simulink model "Target_Control_System"  (R2021b)
settings: Solver=FixedStepDiscrete  StartTime=0.0  StopTime=5  RelTol=1e-3
PreLoadFcn:
  | RTWConfigurationCB('preloadfcn', bdroot);
PostLoadFcn:
  | load('configuration/data_struct.mat');
  | load('configuration/fluxMaps_propMotor.mat');
  | load('configuration/parameterInit_PROP.mat');
  | load('configuration/parameterInit_PUMP.mat');
  | load('configuration/parameterInit_PITCH.mat');
  | load('configuration/parameterInit_TILT.mat');
  | %load('configuration/base_workspace_signal_definition.mat');
  | %load('resolvedatastores_to_baseworkspace_for_faster_simulation.mat');
model workspace (MAT data in the model file):
  SIMULATION_OPTIONS : Simulink.Parameter (value not decoded)
  TARGET_CODE_GEN : Simulink.Parameter (value not decoded)
  TCS_SAMPLE_FREQ_HZ : Simulink.Parameter (value not decoded)
symbols that are objects in the model workspace (value not decoded): TARGET_CODE_GEN, TCS_SAMPLE_FREQ_HZ
undefined symbols (not defined in the file): A_DQ_REF_LPF_INIT__PITCH, A_DQ_REF_LPF_INIT__PROP, A_DQ_REF_LPF_INIT__PUMP, A_DQ_REF_LPF_INIT__TILT, A_OBSERVER_CONFIDENCE_INIT__PITCH, A_OBSERVER_CONFIDENCE_INIT__PROP, A_OBSERVER_CONFIDENCE_INIT__PUMP, A_OBSERVER_CONFIDENCE_INIT__TILT, ACTUATOR_MAX_ANGLE_TRIP__PITCH, ACTUATOR_MIN_ANGLE_TRIP__PITCH, ACTUATOR_POS_SENSOR_INV_DIRECTION__PITCH, ACTUATOR_POS_SENSOR_INV_DIRECTION__TILT, ACTUATOR_POS_SENSOR_OFFSET__PITCH, ACTUATOR_POS_SENSOR_OFFSET__TILT, ADC_scaler1_baseaddr_TILT, ADC_SCALER_FLOAT_TO_FIXPOINT_EXPANSION, ANGLE_ELEC_FROM_SENSOR_OFFSET_INIT__PITCH, ANGLE_ELEC_FROM_SENSOR_OFFSET_INIT__PROP, ANGLE_ELEC_FROM_SENSOR_OFFSET_INIT__PUMP, ANGLE_ELEC_FROM_SENSOR_OFFSET_INIT__TILT, AUTO_CLEAR_FAULTS_ENABLED__PITCH, AUTO_CLEAR_FAULTS_ENABLED__PROP, AUTO_CLEAR_FAULTS_ENABLED__PUMP, AUTO_CLEAR_FAULTS_ENABLED__TILT, AUTO_CLEAR_FAULTS_WAIT_TICKS__PITCH, AUTO_CLEAR_FAULTS_WAIT_TICKS__PROP, AUTO_CLEAR_FAULTS_WAIT_TICKS__PUMP, AUTO_CLEAR_FAULTS_WAIT_TICKS__TILT, AUTO_I_ZERO_IDLE_TICKS__PITCH, AUTO_I_ZERO_IDLE_TICKS__PROP, AUTO_I_ZERO_IDLE_TICKS__PUMP, AUTO_I_ZERO_IDLE_TICKS__TILT, AUTO_I_ZERO_OFFSET_IDC_THRESHOLD__PITCH, AUTO_I_ZERO_OFFSET_IDC_THRESHOLD__PROP, AUTO_I_ZERO_OFFSET_IDC_THRESHOLD__PUMP, AUTO_I_ZERO_OFFSET_IDC_THRESHOLD__TILT, AUTO_I_ZERO_OFFSET_IPH_THRESHOLD__PITCH, AUTO_I_ZERO_OFFSET_IPH_THRESHOLD__PROP, AUTO_I_ZERO_OFFSET_IPH_THRESHOLD__PUMP, AUTO_I_ZERO_OFFSET_IPH_THRESHOLD__TILT, AUTO_SENSORLESS_SWITCHOVER_DISABLE_OMEGA, AUTO_SENSORLESS_SWITCHOVER_ENABLE_OMEGA, AUTO_SENSORLESS_SWITCHOVER_MIN_CONFIDENCE, AUXILIARY_PROTECTION_UNIT_BASEADDR__TILT, blanking_max_error_omega_INIT_PITCH, blanking_max_error_omega_INIT_TILT, blanking_max_error_position_INIT_PITCH, blanking_max_error_position_INIT_TILT, BRUTE_START_I_Q_REF_RAMP_SPEED__PITCH, BRUTE_START_I_Q_REF_RAMP_SPEED__PROP, BRUTE_START_I_Q_REF_RAMP_SPEED__PUMP, BRUTE_START_I_Q_REF_RAMP_SPEED__TILT, CONTROL_LOOP_DT_INIT__PITCH, CONTROL_LOOP_DT_INIT__PROP, CONTROL_LOOP_DT_INIT__PUMP, CONTROL_LOOP_DT_INIT__TILT, CORRECTION_FILTER_SCALE__PITCH, CORRECTION_FILTER_SCALE__PROP, CORRECTION_FILTER_SCALE__PUMP, CORRECTION_FILTER_SCALE__TILT ... (+458)
libraries: simulink x178, Reusables_Lib x24
(part 44 of 47)

== stateflow chart Target_Control_System/MainLoop/tiltMotor_mainLoop/Decimation gate for 10 Hz Tilt/Idle-Loop State Machine Tilt ==
  state InitialState
  state State_90
    //startup delay
    state Wait_Ticks_
    state Startup_Delay_
      entry:
      oTilt.oMot_.oState_.uiDriveState_ = 95;
      oTilt.oMot_.oOut_.uiLastFaultState_ = 0;
    (default) -> State_90.Wait_Ticks_
    State_90.Wait_Ticks_ -> Startup_Delay_ : [after(35, tick)]
  state State_246
    // Second phase of voltage nulling
    state Wait_uiDelayTicks_
    state Next
      entry:
      oTilt.oMot_.oState_.uiDriveState_ = 100;
      oTilt.oMot_.oOut_.uiEnableGateDrive_ = 0x0;
      oTilt.oMot_.oIn_.uiVoltageOffsetNullingActive_ = 0;
    (default) -> State_246.Wait_uiDelayTicks_
    State_246.Wait_uiDelayTicks_ -> State_246.Next : [after(25, tick)]
  state State_95
    // Current offset nulling
    state Wait_Ticks_
    state Current_offset_nulling
      entry:
      oTilt.oMot_.oState_.uiCurrentOffsetNullingPerformed_++;
      oTilt.oMot_.oIn_.uiCurrentOffsetNullingActive_ = 0;
      oTilt.oMot_.oIn_.uiVoltageOffsetNullingActive_ = 0;
      oTilt.oMot_.oState_.uiDriveState_ = 99;
      //SZ: still need to re-write the FPGA protection to enable the sum of current detection for fault 1034
    (default) -> State_95.Wait_Ticks_
    State_95.Wait_Ticks_ -> Current_offset_nulling : [after(6, tick)]
  state State_245
    // Initial phase of voltage nulling
    state Wait_uiDelayTicks_
    state Next
      entry:
      oTilt.oMot_.oState_.uiDriveState_ = 246;
    (default) -> State_245.Wait_uiDelayTicks_
    State_245.Wait_uiDelayTicks_ -> State_245.Next : [after(25, tick)]
  state State_99
    // Minimum command set not met. Also the return state after clearing trips etc.
    state Substate
    state Idle_state
      entry:
      oTilt.oMot_.oState_.uiDriveState_ = 100;
    state Cleanup
      // We somehow left the forced angle start sequence without cleaning up.
      // Clean up now.
      entry:
      oTilt.oMot_.oState_.oRampDataOmegaERef_.oParam_.fUpslope_ = oTilt.oMot_.oState_.fForcedAngleStartOrigOmegaRamp_;
      oTilt.oMot_.oState_.oRampDataOmegaERef_.fSetpoint_ = fabs(oTilt.oMot_.oState_.fForcedAngleStartOrigOmega_);
      oTilt.oMot_.oState_.uiSpeedControllerActive_ = oTilt.oMot_.oState_.uiForcedAngleStartOrigSpeedControllerActive_;
      oTilt.oMot_.oState_.oRampDataIqRef_.oParam_.fUpslope_ = oTilt.oMot_.oState_.fForcedAngleStartOrigIRamp_;
      oTilt.oMot_.oState_.oRampDataIqRef_.oParam_.fDownslope_ = oTilt.oMot_.oState_.oRampDataIqRef_.oParam_.fUpslope_;
      oTilt.oMot_.oOut_.uiForcedAngle_ = 0;
      oTilt.oMot_.oState_.uiForcedAngleStartParametersSet_ = 0;
    (default) -> Substate
    Substate -> (junction 251)
    (junction 251) -> Idle_state [order 2] : [!oTilt.oMot_.oState_.uiMinimumCommandSetFlags_]
    (junction 251) -> State_99.Cleanup [order 1] : [oTilt.oMot_.oState_.uiForcedAngleStartParametersSet_]
    State_99.Cleanup -> Idle_state : [!oTilt.oMot_.oState_.uiMinimumCommandSetFlags_]
  state State_104
    // Idle, motor spinning (windmilling, coasting down),
    // autostart enabled, and a nonzero current applied
    // Removed autostart functionality
    entry:
    oTilt.oMot_.oState_.uiDriveState_ = 102;
  state State_103
    // Idle, motor not spinning, autostart enabled, and a nonzero current applied
    // Removed autostart functionality
    entry:
    oTilt.oMot_.oState_.uiDriveState_ = 101;
  state State_100
    //Idle, determine if the motor is externally driven (e.g. windmilling or spindown) or standing still
    state Initialization
      entry:
      oTilt.oMot_.oState_.oRampDataOmegaERef_.fRampOut_ = 0.0;
      oTilt.oMot_.oState_.oRampDataIqRef_.fRampOut_ = 0.0;
    state Entering_State_101
      entry:
      oTilt.oMot_.oState_.uiDriveState_ = 101;
    state Cleanup
      // We somehow left the forced angle start sequence without cleaning up.
      // Clean up now.
      entry:
      oTilt.oMot_.oState_.uiDriveState_  = 99;
    state Entering_State_102
      entry:
      oTilt.oMot_.oState_.uiDriveState_ = 102;
    state pwm50PercentDuty
      //Pre-set 50% duty
      entry:
      oTilt.oMot_.oOut_.uiPwmRequestFromMain_ = 1;
      oTilt.oMot_.oOut_.uiPwmDutyTicksFromMainA_ = cast(((oTilt.oMot_.oParam_.fPwmPeriodTicksMainloopFloat_) / 2), uint32);
      oTilt.oMot_.oOut_.uiPwmDutyTicksFromMainB_ = cast(((oTilt.oMot_.oParam_.fPwmPeriodTicksMainloopFloat_) / 2), uint32);
      oTilt.oMot_.oOut_.uiPwmDutyTicksFromMainC_ = cast(((oTilt.oMot_.oParam_.fPwmPeriodTicksMainloopFloat_) / 2), uint32);
    (default) -> State_100.Initialization
    State_100.Initialization -> (junction 189)
    (junction 189) -> (junction 186) [order 2]
    (junction 186) -> Entering_State_101 [order 1] : [(fabs(oTilt.oMot_.oOut_.fOmegaEObserverXlpf2_) < oTilt.oMot_.oParam_.fFlyingStartOmegaELimit_) ....
        |  || (oTilt.oMot_.oState_.fObserverConfidence_ < 0.7F)]
    (junction 189) -> State_100.Cleanup [order 1] : [oTilt.oMot_.oState_.uiMinimumCommandSetFlags_]
    (junction 186) -> Entering_State_102 [order 2]
    Entering_State_101 -> pwm50PercentDuty
    Entering_State_102 -> pwm50PercentDuty
  state State_102
    // Idle, motor spinning by external means (windmilling, downhill, large inertia, ....)
    state Stay_at_102
      entry:
      oTilt.oMot_.oState_.uiDriveState_ = 102;
    state Transition_to_101
      entry:
      oTilt.oMot_.oState_.uiDriveState_ = 101;
    (default) -> (junction 192)
    (junction 192) -> Stay_at_102 [order 2]
    (junction 192) -> Transition_to_101 [order 1] : [fabs(oTilt.oMot_.oOut_.fOmegaEObserverXlpf2_) < oTilt.oMot_.oParam_.fFlyingStartOmegaELimit_ ....
        | || oTilt.oMot_.oState_.fObserverConfidence_ < 0.65F]
  state State_101
    // Idle, motor not spinning
    state Initialization
      entry:
      oTilt.oMot_.oState_.oRampDataOmegaERef_.fRampOut_ = 0.0;
      oTilt.oMot_.oState_.oRampDataIqRef_.fRampOut_ = 0.0;
    state Transition_to_102
      entry:
      oTilt.oMot_.oState_.uiDriveState_ = 102;
    (default) -> State_101.Initialization
    State_101.Initialization -> (junction 227)
    (junction 227) -> Transition_to_102 [order 1] : [(fabs(oTilt.oMot_.oOut_.fOmegaEObserverXlpf2_) > oTilt.oMot_.oParam_.fFlyingStartOmegaELimit_) ....
        | && (oTilt.oMot_.oState_.fObserverConfidence_ > 0.65F)]
  (default) -> InitialState
  InitialState -> State_90 [order 1] : [oTilt.oMot_.oState_.uiDriveState_ == 90]
  State_90 -> InitialState : [!(oTilt.oMot_.oState_.uiDriveState_ == 90)]
  InitialState -> State_246 [order 10] : [oTilt.oMot_.oState_.uiDriveState_ == 246]
  State_246 -> InitialState : [!(oTilt.oMot_.oState_.uiDriveState_ == 246)]
  InitialState -> State_95 [order 2] : [oTilt.oMot_.oState_.uiDriveState_ == 95]
  Current_offset_nulling -> InitialState : [!(oTilt.oMot_.oState_.uiDriveState_ == 95)]
  InitialState -> State_245 [order 9] : [oTilt.oMot_.oState_.uiDriveState_ == 245]
  State_245 -> InitialState : [!(oTilt.oMot_.oState_.uiDriveState_ == 245)]
  InitialState -> State_99 [order 3] : [oTilt.oMot_.oState_.uiDriveState_ == 99]
  State_99 -> InitialState : [!(oTilt.oMot_.oState_.uiDriveState_ == 99)]
  InitialState -> State_104 [order 8] : [oTilt.oMot_.oState_.uiDriveState_ == 104]
  State_104 -> InitialState
  InitialState -> State_103 [order 7] : [oTilt.oMot_.oState_.uiDriveState_ == 103]
  State_103 -> InitialState
  InitialState -> State_102 [order 6] : [oTilt.oMot_.oState_.uiDriveState_ == 102]
  Stay_at_102 -> InitialState
  State_100.Cleanup -> InitialState
  Transition_to_101 -> InitialState
  pwm50PercentDuty -> InitialState
  InitialState -> State_100 [order 4] : [oTilt.oMot_.oState_.uiDriveState_ == 100]
  InitialState -> State_101 [order 5] : [oTilt.oMot_.oState_.uiDriveState_ == 101]
  (junction 227) -> InitialState [order 2] : // We're staying at rest.
  Transition_to_102 -> InitialState
  data: oTilt data_store_memory; PI_F constant single =3.14159265359; TWO_PI_F constant single =6.28318530718

== stateflow chart Target_Control_System/MainLoop/pitchMotor_mainLoop/Decimation gate for 200 Hz Pitch/Function-Call Subsystem/Check zero current if inverter off/Enabled Subsystem/Chart ==
  state Start
  state Drive_trip
    // Disable the drive and enter a trip state (error state)
    entry:
    oPitch.oMot_.oOut_.uiEnableGateDrive_ = 0;
    oPitch.oMot_.oOut_.uiCurrentControllerActive_ = 0;
    // NOTE: the actual turning off is done in the ctrl interrupt
    // formerly: Xil_Out32(uiGateDriverBaseaddr_, 0x0);
  state Store_previous_fault
    // If we were already in a fault state, store the previous fault:
    entry:
    oPitch.oMot_.oOut_.uiLastFaultState_ = oPitch.oMot_.oState_.uiDriveState_;
  state setTripState
    entry:
    oPitch.oMot_.oState_.uiDriveState_ = 1042;
  (default) -> Start
  setTripState -> Start
  Start -> (junction 14) : [fabs(oPitch.oMot_.oIn_.oAdcData_.fIa_) > oPitch.oMot_.oParam_.fMaximumPhaseCurrentWhileOff_ || ...
      | fabs(oPitch.oMot_.oIn_.oAdcData_.fIb_) > oPitch.oMot_.oParam_.fMaximumPhaseCurrentWhileOff_ || ...
      | fabs(oPitch.oMot_.oIn_.oAdcData_.fIc_) > oPitch.oMot_.oParam_.fMaximumPhaseCurrentWhileOff_]
  (junction 14) -> Drive_trip [order 1] : [oPitch.oMot_.oState_.uiDriveState_ >= 200]
  (junction 14) -> (junction 19) [order 2]
  Drive_trip -> (junction 19)
  (junction 19) -> Store_previous_fault [order 1] : [oPitch.oMot_.oState_.uiDriveState_ >= 1000]
  (junction 19) -> setTripState [order 2]
  Store_previous_fault -> setTripState
  data: oPitch data_store_memory

== stateflow chart Target_Control_System/MainLoop/pitchMotor_mainLoop/Decimation gate for 200 Hz Pitch/Function-Call Subsystem/Current offset nulling/initiateOffsetNulling(&oPitch)/Chart ==
  state Start
  state initiateOffsetNulling
    //We can only do this if idle
    entry:
    oPitch.oIsr_.oState_.fOffsetIntegratorIa_ = 0.0;
    oPitch.oIsr_.oState_.fOffsetIntegratorIb_ = 0.0;
    oPitch.oIsr_.oState_.fOffsetIntegratorIc_ = 0.0;
    oPitch.oIsr_.oState_.fOffsetIntegratorIdc_ = 0.0;
    oPitch.oMot_.oState_.uiDriveState_ = 95;
  (default) -> Start
  initiateOffsetNulling -> Start : [oPitch.oMot_.oState_.uiCurrentOffsetNullingPerformed_ == 1]
  Start -> initiateOffsetNulling : [oPitch.oMot_.oState_.uiDriveState_ >= 99 && ...
      | oPitch.oMot_.oState_.uiDriveState_ < 102]
  data: oPitch data_store_memory

== stateflow chart Target_Control_System/MainLoop/tiltMotor_mainLoop/Decimation gate for 10 Hz Tilt/Function-Call Subsystem/DC_overvoltage ==
  state Start
  state Drive_trip
    // Disable the drive and enter a trip state (error state)
    entry:
    oTilt.oMot_.oOut_.uiEnableGateDrive_ = 0;
    oTilt.oMot_.oOut_.uiCurrentControllerActive_ = 0;
    // NOTE: the actual turning off is done in the ctrl interrupt
    // formerly: Xil_Out32(uiGateDriverBaseaddr_, 0x0);
  state Store_previous_fault
    // If we were already in a fault state, store the previous fault:
    entry:
    oTilt.oMot_.oOut_.uiLastFaultState_ = oTilt.oMot_.oState_.uiDriveState_;
  state setTripState
    entry:
    oTilt.oMot_.oState_.uiDriveState_ = Udc_tripCode;
  (default) -> Start
  Start -> (junction 10) [order 2] : [(oTilt.oMot_.oOut_.fUdcLpf_ > oTilt.oMot_.oParam_.fUdcMaxTrip_) && ...
      | oTilt.oMot_.oState_.uiDriveState_ > 0]
      | {Udc_tripCode = 1004;}
  Start -> (junction 10) [order 1] : [oTilt.oMot_.oOut_.fUdcLpf_ < oTilt.oMot_.oParam_.fUdcMinTrip_ && ...
      | (oTilt.oMot_.oState_.uiDriveState_ > 199 && oTilt.oMot_.oState_.uiDriveState_ < 1000)]
      | {Udc_tripCode = 1003;}
  setTripState -> Start
  (junction 10) -> Drive_trip [order 1] : [oTilt.oMot_.oState_.uiDriveState_ >= 200]
  (junction 10) -> (junction 18) [order 2]
  Drive_trip -> (junction 18)
  (junction 18) -> Store_previous_fault [order 1] : [oTilt.oMot_.oState_.uiDriveState_ >= 1000]
  (junction 18) -> setTripState [order 2]
  Store_previous_fault -> setTripState
  data: Udc_tripCode local single; oTilt data_store_memory

== stateflow chart Target_Control_System/MainLoop/pitchMotor_mainLoop/mainTask_pitch/motorTaskMainFastStep()/Software Overcurrent Protection - Pitch/Forced_angle_overcurrent/Chart ==
  state Start
    // During forced angle start use a lower overcurrent limit, because we know exactly how much current should flow in the motor
    entry:
    fMaximumCurrent = oPitch.oMot_.oParam_.fForcedAngleIRef_ * oPitch.oMot_.oParam_.fForcedAngleStartOvercurrentRatio_;
  state Drive_trip
    // Disable the drive and enter a trip state (error state)
    entry:
    oPitch.oMot_.oOut_.uiEnableGateDrive_ = 0;
    oPitch.oMot_.oOut_.uiCurrentControllerActive_ = 0;
    // NOTE: the actual turning off is done in the ctrl interrupt
    // formerly: Xil_Out32(uiGateDriverBaseaddr_, 0x0);
  state Store_previous_fault
    // If we were already in a fault state, store the previous fault:
    entry:
    oPitch.oMot_.oOut_.uiLastFaultState_ = oPitch.oMot_.oState_.uiDriveState_;
  state setTripState
    entry:
    oPitch.oMot_.oState_.uiDriveState_ = 1041;
  (default) -> Start
  Start -> (junction 7) : [single(fabs(oPitch.oMot_.oIn_.oAdcData_.fIa_)) > fMaximumCurrent || ...
      | single(fabs(oPitch.oMot_.oIn_.oAdcData_.fIb_)) > fMaximumCurrent || ...
      | single(fabs(oPitch.oMot_.oIn_.oAdcData_.fIc_)) > fMaximumCurrent]
  setTripState -> Start
  (junction 7) -> Drive_trip [order 1] : [oPitch.oMot_.oState_.uiDriveState_ >= 200]
  (junction 7) -> (junction 14) [order 2]
  Drive_trip -> (junction 14)
  (junction 14) -> Store_previous_fault [order 1] : [oPitch.oMot_.oState_.uiDriveState_ >= 1000]
  (junction 14) -> setTripState [order 2]
  Store_previous_fault -> setTripState
  data: oPitch data_store_memory; fMaximumCurrent local double

== stateflow chart Target_Control_System/MainLoop/pitchMotor_mainLoop/mainTask_pitch/motorTaskMainFastStep()/Software Overcurrent Protection - Pitch/checkForHwOvercurrents(&oPitch)/checkForHwOvercurrents  ==
  state Start
  state setTripState3
    //default aux trip
    entry:
    oPitch.oMot_.oState_.uiDriveState_ = 1018;
  state Drive_trip1
    // Disable the drive and enter a trip state (error state)
    entry:
    oPitch.oMot_.oOut_.uiEnableGateDrive_ = 0;
    oPitch.oMot_.oOut_.uiCurrentControllerActive_ = 0;
    // NOTE: the actual turning off is done in the ctrl interrupt
    // formerly: Xil_Out32(uiGateDriverBaseaddr_, 0x0);
  state Store_previous_fault3
    // If we were already in a fault state, store the previous fault:
    entry:
    oPitch.oMot_.oOut_.uiLastFaultState_ = oPitch.oMot_.oState_.uiDriveState_;
  state Store_previous_fault1
    // If we were already in a fault state, store the previous fault:
    entry:
    oPitch.oMot_.oOut_.uiLastFaultState_ = oPitch.oMot_.oState_.uiDriveState_;
  state Drive_trip3
    // Disable the drive and enter a trip state (error state)
    entry:
    oPitch.oMot_.oOut_.uiEnableGateDrive_ = 0;
    oPitch.oMot_.oOut_.uiCurrentControllerActive_ = 0;
    // NOTE: the actual turning off is done in the ctrl interrupt
    // formerly: Xil_Out32(uiGateDriverBaseaddr_, 0x0);
  state setTripState1
    // Hardware overcurrent trip
    entry:
    oPitch.oMot_.oState_.uiDriveState_ = 1008;
  state Aux_trip
    // Auxiliary trip, one-hot encoding in bits 6:4
    entry:
    oPitch.oMot_.oOut_.uiGateDriverStatus_ &= 0x70;
    fTemp = oPitch.oMot_.oOut_.uiGateDriverStatus_ >> 4;
    oPitch.oMot_.oOut_.uiGateDriverStatus_ = fTemp;
  state Drive_trip2
    // Disable the drive and enter a trip state (error state)
    entry:
    oPitch.oMot_.oOut_.uiEnableGateDrive_ = 0;
    oPitch.oMot_.oOut_.uiCurrentControllerActive_ = 0;
    // NOTE: the actual turning off is done in the ctrl interrupt
    // formerly: Xil_Out32(uiGateDriverBaseaddr_, 0x0);
  state Aux_trip_2
    // Aux trip 2: The hardware monitor for the control voltages has tripped.
    // This circuit is not present on the January 2019 inverters, but the FPGA image holds
    // the lines at the non-tripped levels.
    // Some of the GPIO pins will tell us which voltage rail tripped:
    entry:
    fTemp2 = mdl_pitch_uiFlags & 0x1F;
    fTemp2 ^= 0x4;
    mdl_pitch_uiFlags = fTemp2;
    //3V = 1036; 5V = 1037; 12V = 1038; default = 1039 (more than one control voltage low simultaneously);
  state Store_previous_fault2
    // If we were already in a fault state, store the previous fault:
    entry:
    oPitch.oMot_.oOut_.uiLastFaultState_ = oPitch.oMot_.oState_.uiDriveState_;
  state Drive_trip5
    // Disable the drive and enter a trip state (error state)
    entry:
    oPitch.oMot_.oOut_.uiEnableGateDrive_ = 0;
    oPitch.oMot_.oOut_.uiCurrentControllerActive_ = 0;
    // NOTE: the actual turning off is done in the ctrl interrupt
    // formerly: Xil_Out32(uiGateDriverBaseaddr_, 0x0);
  state setTripState2
    //Aux trip 1: software watchdog timer
    entry:
    oPitch.oMot_.oState_.uiDriveState_ = 1015;
  state Store_previous_fault5
    // If we were already in a fault state, store the previous fault:
    entry:
    oPitch.oMot_.oOut_.uiLastFaultState_ = oPitch.oMot_.oState_.uiDriveState_;
  state Drive_trip4
    // Disable the drive and enter a trip state (error state)
    entry:
    oPitch.oMot_.oOut_.uiEnableGateDrive_ = 0;
    oPitch.oMot_.oOut_.uiCurrentControllerActive_ = 0;
    // NOTE: the actual turning off is done in the ctrl interrupt
    // formerly: Xil_Out32(uiGateDriverBaseaddr_, 0x0);
  state setTripState5
    entry:
    oPitch.oMot_.oState_.uiDriveState_ = aux3_tripCode;
  state Store_previous_fault4
    // If we were already in a fault state, store the previous fault:
    entry:
    oPitch.oMot_.oOut_.uiLastFaultState_ = oPitch.oMot_.oState_.uiDriveState_;
  state setTripState4
    //Aux trip 1: software watchdog timer
    entry:
    oPitch.oMot_.oState_.uiDriveState_ = aux2_tripCode;
  (default) -> Start
  setTripState4 -> Start
  setTripState2 -> Start
  setTripState3 -> Start
  Start -> Aux_trip [order 2] : [(oPitch.oMot_.oOut_.uiGateDriverStatus_ & 0x70) > 0]
  Start -> (junction 20) [order 1] : [(oPitch.oMot_.oOut_.uiGateDriverStatus_ & 0xE) > 0]
  setTripState1 -> Start
  setTripState5 -> Start
  (junction 20) -> Drive_trip1 [order 1] : [oPitch.oMot_.oState_.uiDriveState_ >= 200]
  Store_previous_fault3 -> setTripState3
  (junction 64) -> setTripState3 [order 2]
  (junction 20) -> (junction 25) [order 2]
  Drive_trip1 -> (junction 25)
  (junction 64) -> Store_previous_fault3 [order 1] : [oPitch.oMot_.oState_.uiDriveState_ >= 1000]
  Drive_trip3 -> (junction 64)
  (junction 57) -> (junction 64) [order 2]
  (junction 25) -> Store_previous_fault1 [order 1] : [oPitch.oMot_.oState_.uiDriveState_ >= 1000]
  (junction 25) -> setTripState1 [order 2]
  Store_previous_fault1 -> setTripState1
  (junction 57) -> Drive_trip3 [order 1] : [oPitch.oMot_.oState_.uiDriveState_ >= 200]
  Aux_trip -> (junction 57) [order 4]
  Aux_trip -> (junction 40) [order 3] : [fTemp == 1]
  Aux_trip -> Aux_trip_2 [order 2] : [fTemp == 2]
      | // C code uses oPitch.oMot_.oOut_.uiGateDriverStatus_ == 2, but this value gets rewritten
      | // at each time step so it doesn't work for stateflow transition.
  Aux_trip -> (junction 170) [order 1] : [fTemp == 4]
      | // Aux Trip 3. This is the auxiliary protection unit.
      | // If this is a known error, set that specific fault code.
  (junction 40) -> Drive_trip2 [order 1] : [oPitch.oMot_.oState_.uiDriveState_ >= 200]
  (junction 40) -> (junction 48) [order 2]
  Drive_trip2 -> (junction 48)
  Aux_trip_2 -> (junction 85) [order 1] : [fTemp2 == 1]
      | {aux2_tripCode = 1036;}
  Aux_trip_2 -> (junction 85) [order 2] : [fTemp2 == 2 || ...
      | fTemp2 == 8]
      | {aux2_tripCode = 1037;}
  Aux_trip_2 -> (junction 85) [order 3] : [fTemp2 == 4 || ...
      | fTemp2 == 16]
      | {aux2_tripCode = 1038;}
  Aux_trip_2 -> (junction 85) [order 4] : {aux2_tripCode = 1039;}
  (junction 48) -> Store_previous_fault2 [order 1] : [oPitch.oMot_.oState_.uiDriveState_ >= 1000]
  (junction 48) -> setTripState2 [order 2]
  (junction 170) -> (junction 150) [order 3] : {aux3_tripCode = 1017;}
  Store_previous_fault2 -> setTripState2
  (junction 170) -> (junction 150) [order 2] : [mdl_pitch_uiAPUFlags == 2]
      | {aux3_tripCode = 1035;}
      | // Digitally stuck sensor
  (junction 150) -> Drive_trip5 [order 1] : [oPitch.oMot_.oState_.uiDriveState_ >= 200]
  (junction 170) -> (junction 150) [order 1] : [mdl_pitch_uiAPUFlags == 1]
      | {aux3_tripCode = 1034;}
      | // Phase current sum out of bounds.
      | // This could happen at boot due to offsets.
      | // If this is indeed the case, this fault may
      | // need to be ignored until current zeroing
      | // has been done. For now, keep it simple.
  (junction 150) -> (junction 159) [order 2]
  Drive_trip5 -> (junction 159)
  (junction 159) -> Store_previous_fault5 [order 1] : [oPitch.oMot_.oState_.uiDriveState_ >= 1000]
  (junction 159) -> setTripState5 [order 2]
  (junction 85) -> Drive_trip4 [order 1] : [oPitch.oMot_.oState_.uiDriveState_ >= 200]
  (junction 85) -> (junction 103) [order 2]
  Store_previous_fault5 -> setTripState5
  Drive_trip4 -> (junction 103)
  (junction 103) -> Store_previous_fault4 [order 1] : [oPitch.oMot_.oState_.uiDriveState_ >= 1000]
  (junction 103) -> setTripState4 [order 2]
  Store_previous_fault4 -> setTripState4
  data: aux2_tripCode local single; fTemp local uint32; oPitch data_store_memory; mdl_pitch_uiFlags data_store_memory; aux3_tripCode local double; mdl_pitch_uiAPUFlags data_store_memory; fTemp2 local double

== stateflow chart Target_Control_System/MainLoop/pitchMotor_mainLoop/mainTask_pitch/motorTaskMainFastStep()/Software Overcurrent Protection - Pitch/softwareOvercurrentProtection ==
  state Start
  state Drive_trip
    // Disable the drive and enter a trip state (error state)
    entry:
    oPitch.oMot_.oOut_.uiEnableGateDrive_ = 0;
    oPitch.oMot_.oOut_.uiCurrentControllerActive_ = 0;
    // NOTE: the actual turning off is done in the ctrl interrupt
    // formerly: Xil_Out32(uiGateDriverBaseaddr_, 0x0);
  state Store_previous_fault
    // If we were already in a fault state, store the previous fault:
    entry:
    oPitch.oMot_.oOut_.uiLastFaultState_ = oPitch.oMot_.oState_.uiDriveState_;
  state setTripState
    entry:
    oPitch.oMot_.oState_.uiDriveState_ = 1007;
  (default) -> Start
  Start -> (junction 7) : [oPitch.oMot_.oIn_.fIPhaseMagnitude_ > oPitch.oMot_.oParam_.fTripLimitSoftwareA_]
  (junction 7) -> Drive_trip [order 1] : [oPitch.oMot_.oState_.uiDriveState_ >= 200]
  (junction 7) -> (junction 10) [order 2]
  Drive_trip -> (junction 10)
  (junction 10) -> Store_previous_fault [order 1] : [oPitch.oMot_.oState_.uiDriveState_ >= 1000]
  (junction 10) -> setTripState [order 2]
  Store_previous_fault -> setTripState
  data: oPitch data_store_memory

== stateflow chart Target_Control_System/MainLoop/pitchMotor_mainLoop/mainTask_pitch/motorTaskMainFastStep()/enableDrive(&oPitch) ==
  state Disabled
    state Default
    state Disable_Drive
      entry:
      oPitch.oMot_.oState_.uiDriveState_ = 100;
      oPitch.oMot_.oOut_.uiEnableGateDrive_ = 0x0;
      oPitch.oMot_.oOut_.uiCurrentControllerActive_ = 0;
    state Simulation
      entry:
      oPitch.oMot_.oState_.uiDriveState_ = 101;
      oPitch.oMot_.oOut_.uiEnableGateDrive_ = 0x0;
    (default) -> (junction 289)
    (junction 289) -> Default [order 3]
    (junction 289) -> Disable_Drive [order 2] : [oPitch.oMot_.oState_.uiDriveState_ >= 200 && ....
        |  oPitch.oMot_.oState_.uiDriveState_ <= 299]
    (junction 289) -> Simulation [order 1] : [TARGET_CODE_GEN ==0]
  state Position_hold_mode
    // Mostly intended for the VP. In position hold mode, the inverter will inject 0 RPM current in the motor to passively hold a motor in place.
    // The position sensors are not needed for this.
    // When issuing the enable command, the drive enters state 226, which is just for flagging, the inverters do not actually turn on.
    // (Use a special command for that.)
    entry:
    oPitch.oMot_.oState_.uiDriveState_ = 226;
    oPitch.oIsr_.oParam_.oPiDataIq_.fState_ = 0;
    oPitch.oIsr_.oParam_.oPiDataId_.fState_ = 0;
    // Pre-set 50% duty
    oPitch.oMot_.oOut_.uiPwmRequestFromMain_ = 1;
    oPitch.oMot_.oOut_.uiPwmDutyTicksFromMainA_ = uint32((oPitch.oMot_.oParam_.fPwmPeriodTicksMainloopFloat_)/2);
    oPitch.oMot_.oOut_.uiPwmDutyTicksFromMainB_ = uint32((oPitch.oMot_.oParam_.fPwmPeriodTicksMainloopFloat_)/2);
    oPitch.oMot_.oOut_.uiPwmDutyTicksFromMainC_ = uint32((oPitch.oMot_.oParam_.fPwmPeriodTicksMainloopFloat_)/2);
  state DC_undervoltage_trip
    state Fault_A
      entry:
      oPitch.oMot_.oOut_.uiCurrentControllerActive_ = 0;
      oPitch.oMot_.oOut_.uiEnableGateDrive_ = 0;
    state Fault_B
      // If we were already in a fault state, store the previous fault:
      entry:
      oPitch.oMot_.oOut_.uiLastFaultState_ = oPitch.oMot_.oState_.uiDriveState_;
    state Fault_C
      entry:
      oPitch.oMot_.oState_.uiDriveState_ = 1003;
    (default) -> (junction 164)
    (junction 164) -> Fault_A [order 1] : [oPitch.oMot_.oState_.uiDriveState_>= 200]
    (junction 164) -> (junction 271) [order 2]
    (junction 271) -> Fault_C [order 2]
    (junction 271) -> Fault_B [order 1] : [oPitch.oMot_.oState_.uiDriveState_>= 1000]
    Fault_B -> Fault_C
  state Slave_start
    // Slave start is not applicable to position control.
    // Not a position control inverter; slave role is set: Perform a slave start (wait for the motor to 'somehow' reach a minimum speed, then jump on).
    entry:
    // We have to set one item aside; the desired rotation direction, as signalled by the sign of the current
    oPitch.oMot_.oState_.fForcedAngleStartDirection_ = single(oPitch.oMot_.oIn_.fIqSetpoint_ >= 0);
    // in other areas of MBD, we use oPitch.oMot_.oState_.oRampDataIqRef_.fRampOut_...should we here?
    // Don't actually turn on the output stage, but instead, monitor the motor feedback.
    // Once confident, perform a running start.
    // The rest is handled via state machine.
    oPitch.oMot_.oState_.uiDriveState_ = 220;
  state Enabled
    // [SZ]: Still need to model the setupForFlyingStart() function, which involves calling NEON sin/cos functions in Stateflow
    state Open_loop_start
      // Open loop start from standstill. Risky, and rough on hardware
      state Open_loop_start_A
        entry:
        oPitch.oMot_.oState_.oRampDataFluxFeedforwardGain_.fRampOut_ = 0.0;
        oPitch.oMot_.oState_.oRampDataOmegaERef_.fRampOut_ = 0.0;
        oPitch.oMot_.oState_.oRampDataIqRef_.fRampOut_ = 0.0;
        oPitch.oMot_.oState_.uiDriveState_ = 200;
      state Open_loop_start_B
        entry:
        oPitch.oMot_.oState_.uiDriveState_ = 205;
      (default) -> Open_loop_start_A
      Open_loop_start_A -> Open_loop_start_B [order 1] : [oPitch.oMot_.oParam_.uiAutomaticFanControlMode_ == 1]
    state Standing_start
      // ----- Set up for forced angle start ----
      state Store_reference
        // Store original references and ramp rates aside:
        entry:
        oPitch.oMot_.oState_.fForcedAngleStartOrigIRamp_ = oPitch.oMot_.oState_.oRampDataIqRef_.oParam_.fUpslope_;
        // TODO: whatabout downslope?
        oPitch.oMot_.oState_.fForcedAngleStartOrigOmega_ = oPitch.oMot_.oState_.oRampDataOmegaERef_.fSetpoint_;
        oPitch.oMot_.oState_.fForcedAngleStartOrigOmegaRamp_ = oPitch.oMot_.oState_.oRampDataOmegaERef_.oParam_.fUpslope_;
        // The downslope is never touched, as it doesn't matter for forced angle start
        oPitch.oMot_.oState_.uiForcedAngleStartOrigSpeedControllerActive_ = oPitch.oMot_.oState_.uiSpeedControllerActive_;
        // We have to set one item aside; the desired rotation direction, as signalled by the sign of the current
        oPitch.oMot_.oState_.fForcedAngleStartDirection_ = single(oPitch.oMot_.oState_.oRampDataIqRef_.fRampOut_ >= 0);
        // should this be oPitch.oMot_.oIn_.fIqSetpoint_ >= 0; ??
      state Global_signal
        // Signals to the rest of the program.
        oPitch.oMot_.oOut_.uiForcedAngle_ = 1;
        oPitch.oMot_.oState_.uiDriveState_ = 211;
      state Initialization
        // Set up initial values
        entry:
        // Delete this section once the uiForcedAngleStartParametersSet_ flag is working properly...
        oPitch.oMot_.oState_.fForcedAngleStartOrigIRamp_ = oPitch.oMot_.oState_.oRampDataIqRef_.oParam_.fUpslope_;
        // TODO: whatabout downslope?
        oPitch.oMot_.oState_.fForcedAngleStartOrigOmega_ = oPitch.oMot_.oState_.oRampDataOmegaERef_.fSetpoint_;
        oPitch.oMot_.oState_.fForcedAngleStartOrigOmegaRamp_ = oPitch.oMot_.oState_.oRampDataOmegaERef_.oParam_.fUpslope_;
        // The downslope is never touched, as it doesn't matter for forced angle start
        oPitch.oMot_.oState_.uiForcedAngleStartOrigSpeedControllerActive_ = oPitch.oMot_.oState_.uiSpeedControllerActive_;
        // We have to set one item aside; the desired rotation direction, as signalled by the sign of the current
        oPitch.oMot_.oState_.fForcedAngleStartDirection_ = single(oPitch.oMot_.oState_.oRampDataIqRef_.fRampOut_ >= 0);
        oPitch.oMot_.oState_.fIqRefBeforeRamp_ = oPitch.oMot_.oParam_.fForcedAngleIRef_;
        //oPitch.oMot_.oState_.oRampDataIqRef_.oParam_.fUpslope_ = oPitch.oMot_.oParam_.fForcedAngleIRamp_;
        oPitch.oMot_.oState_.oRampDataIqRef_.oParam_.fUpslope_ = oPitch.oMot_.oParam_.fForcedAngleIRamp_*10*(TARGET_CODE_GEN==0)+...
        oPitch.oMot_.oParam_.fForcedAngleIRamp_*(TARGET_CODE_GEN==1); // Adjust for 100 Hz state machine in simulation
        oPitch.oMot_.oState_.oRampDataIqRef_.oParam_.fDownslope_ = oPitch.oMot_.oState_.oRampDataIqRef_.oParam_.fUpslope_;
        //oPitch.oMot_.oState_.oRampDataOmegaERef_.oParam_.fUpslope_ = oPitch.oMot_.oParam_.fForcedAngleOmegaERamp_;
        oPitch.oMot_.oState_.oRampDataOmegaERef_.oParam_.fUpslope_ = oPitch.oMot_.oParam_.fForcedAngleOmegaERamp_*10*(TARGET_CODE_GEN==0)+...
        oPitch.oMot_.oParam_.fForcedAngleOmegaERamp_*(TARGET_CODE_GEN==1); // Adjust for 100 Hz state machine in simulation
        oPitch.oMot_.oState_.oRampDataOmegaERef_.fRampOut_ = 0.0F;
        oPitch.oMot_.oState_.oRampDataOmegaERef_.fSetpoint_ = 0.0F;
        oPitch.oMot_.oState_.oRampDataIqRef_.fRampOut_ = 0.0F;
        oPitch.oMot_.oState_.uiSpeedControllerActive_ = 0;
        oPitch.oMot_.oState_.uiForcedAngleStartParametersSet_ = 1;
        oPitch.oMot_.oState_.oRampDataFluxFeedforwardGain_.fRampOut_ = 0.0F;
      (default) -> Global_signal
      Global_signal -> (junction 233)
      (junction 233) -> Store_reference [order 1] : [!(oPitch.oMot_.oState_.uiForcedAngleStartParametersSet_ == 1)]
      (junction 233) -> Initialization [order 2]
      Store_reference -> Initialization
    state Half_duty_preset
      // Pre-set 50% duty
      entry:
      oPitch.oMot_.oOut_.uiPwmRequestFromMain_ = 1;
      oPitch.oMot_.oOut_.uiPwmDutyTicksFromMainA_ = uint32((oPitch.oMot_.oParam_.fPwmPeriodTicksMainloopFloat_)/2);
      oPitch.oMot_.oOut_.uiPwmDutyTicksFromMainB_ = uint32((oPitch.oMot_.oParam_.fPwmPeriodTicksMainloopFloat_)/2);
      oPitch.oMot_.oOut_.uiPwmDutyTicksFromMainC_ = uint32((oPitch.oMot_.oParam_.fPwmPeriodTicksMainloopFloat_)/2);
      oPitch.oIsr_.oParam_.oPiDataIq_.fState_ = 0.0F;
      oPitch.oIsr_.oParam_.oPiDataId_.fState_ = 0.0F;
      oPitch.oMot_.oParam_.oPiDataRpm_.fState_ = 0.0F;
      oPitch.oMot_.oParam_.oPid2DataRpmCtrl_.fState_ = 0.0F;
      oPitch.oMot_.oState_.oPosSensor_.oPidDataPosCtrl_.fState_ = 0.0F;
      oPitch.oMot_.oState_.oRampDataPos_.fRampOut_ = oPitch.oMot_.oState_.oPosSensor_.oGbx_.fCurrentOutputAngle_;
      // Prevent jerk motions on start up.
      // [SZ]: Moved here to avoid the "Unconditional Path Out of State with During Actions or Child States" warning
    state Release_gate_signal
      entry:
      oPitch.oIsr_.oState_.fOverspeedProtectionScaler_ = 1.0;
      oPitch.oMot_.oState_.oPosSensor_.iAngleElecFromSensorNumOfIdenticalValues_ = 0;
      // release gate signals
      oPitch.oMot_.oOut_.uiEnableGateDrive_ = 0x7;
      oPitch.oMot_.oOut_.uiCurrentControllerActive_ = 1; // Release control in main interrupt
    (default) -> (junction 184)
    (junction 184) -> Open_loop_start [order 2]
    (junction 184) -> Standing_start [order 1] : [oPitch.oMot_.oState_.uiForcedAngleStart_ == 1]
    Open_loop_start_A -> Half_duty_preset [order 2]
    Open_loop_start_B -> Half_duty_preset
    Initialization -> Half_duty_preset
    Half_duty_preset -> Release_gate_signal
  (default) -> Disabled
  Slave_start -> Disabled
  Position_hold_mode -> Disabled
  (junction 192) -> Disabled [order 1] : [oPitch.oMot_.oState_.uiDriveState_ < 101 || oPitch.oMot_.oState_.uiDriveState_ > 104]
  Disabled -> (junction 192) : [oPitch.oMot_.oOut_.uiEnable_ == 1]
  DC_undervoltage_trip -> Disabled : [oPitch.oMot_.oOut_.fUdcLpf_ > oPitch.oMot_.oParam_.fUdcMinTrip_]
  Enabled -> Disabled : [!(oPitch.oMot_.oOut_.uiEnable_ == 1)]
  (junction 192) -> Position_hold_mode [order 3] : [oPitch.oMot_.oParam_.iForcedPositionHoldMode_ == 1]
  (junction 192) -> DC_undervoltage_trip [order 2] : [oPitch.oMot_.oOut_.fUdcLpf_< oPitch.oMot_.oParam_.fUdcMinTrip_]
  (junction 192) -> Slave_start [order 4] : [oPitch.oMot_.oParam_.uiSlaveRole_ == 1 && !(oPitch.oMot_.oState_.oPosSensor_.iPosControlEnabled_ == 1)]
  (junction 192) -> (junction 273) [order 5]
  (junction 273) -> Enabled : [oPitch.oMot_.oState_.uiDriveState_ == 101 || oPitch.oMot_.oState_.uiDriveState_ == 103]
  data: TARGET_CODE_GEN parameter; oPitch data_store_memory

== stateflow chart Target_Control_System/MainLoop/propMotor_mainLoop/Decimation gate A for 200 Hz Prop/Cross-tripping VP//Tilt to Prop/VP to Prop ==
  state Start
  state Drive_trip
    // Disable the drive and enter a trip state (error state)
    entry:
    oProp.oMot_.oOut_.uiEnableGateDrive_ = 0;
    oProp.oMot_.oOut_.uiCurrentControllerActive_ = 0;
    // NOTE: the actual turning off is done in the ctrl interrupt
    // formerly: Xil_Out32(uiGateDriverBaseaddr_, 0x0);
  state Store_previous_fault
    // If we were already in a fault state, store the previous fault:
    entry:
    oProp.oMot_.oOut_.uiLastFaultState_ = oProp.oMot_.oState_.uiDriveState_;
  state setTripState
    entry:
    oProp.oMot_.oState_.uiDriveState_ = 1028;
  (default) -> Start
  (junction 40) -> Start [order 2]
  Start -> (junction 19) : [iCrossTripPitchToPropulsionMode > 0]
  (junction 21) -> Start [order 2]
  (junction 26) -> Start [order 2]
  setTripState -> Start
  (junction 19) -> (junction 40) [order 2]
  (junction 40) -> (junction 42) [order 1] : [oPitch.oMot_.oState_.uiDriveState_ != 200]
  (junction 19) -> (junction 21) [order 1] : [iCrossTripPitchToPropulsionMode == 2]
  (junction 21) -> (junction 26) [order 1] : [oPitch.oMot_.oState_.uiDriveState_ >= 1000]
  (junction 42) -> (junction 26)
  (junction 26) -> (junction 27) [order 1] : [oProp.oMot_.oState_.uiDriveState_ >= 200 && oProp.oMot_.oState_.uiDriveState_ < 300]
  (junction 27) -> Drive_trip [order 1] : [oProp.oMot_.oState_.uiDriveState_ >= 200]
  (junction 27) -> (junction 35) [order 2]
  Drive_trip -> (junction 35)
  (junction 35) -> Store_previous_fault [order 1] : [oProp.oMot_.oState_.uiDriveState_ >= 1000]
  (junction 35) -> setTripState [order 2]
  data: oProp data_store_memory; oPitch data_store_memory; iCrossTripPitchToPropulsionMode data_store_memory

== stateflow chart Target_Control_System/MainLoop/propMotor_mainLoop/Decimation gate A for 200 Hz Prop/Cross-tripping VP//Tilt to Prop/Tilt to Prop ==
  state Start
  state Drive_trip
    // Disable the drive and enter a trip state (error state)
    entry:
    oProp.oMot_.oOut_.uiEnableGateDrive_ = 0;
    oProp.oMot_.oOut_.uiCurrentControllerActive_ = 0;
    // NOTE: the actual turning off is done in the ctrl interrupt
    // formerly: Xil_Out32(uiGateDriverBaseaddr_, 0x0);
  state Store_previous_fault
    // If we were already in a fault state, store the previous fault:
    entry:
    oProp.oMot_.oOut_.uiLastFaultState_ = oProp.oMot_.oState_.uiDriveState_;
  state setTripState
    entry:
    oProp.oMot_.oState_.uiDriveState_ = 1027;
  (default) -> Start
  (junction 40) -> Start [order 2]
  Start -> (junction 19) : [iCrossTripTiltToPropulsionMode > 0]
  (junction 21) -> Start [order 2]
  (junction 26) -> Start [order 2]
  setTripState -> Start
  (junction 19) -> (junction 40) [order 2]
  (junction 40) -> (junction 42) [order 1] : [oTilt.oMot_.oState_.uiDriveState_ != 200]
  (junction 19) -> (junction 21) [order 1] : [iCrossTripTiltToPropulsionMode == 2]
  (junction 21) -> (junction 26) [order 1] : [oTilt.oMot_.oState_.uiDriveState_ >= 1000]
  (junction 42) -> (junction 26)
  (junction 26) -> (junction 27) [order 1] : [oProp.oMot_.oState_.uiDriveState_ >= 200 && oProp.oMot_.oState_.uiDriveState_ < 300]
  (junction 27) -> Drive_trip [order 1] : [oProp.oMot_.oState_.uiDriveState_ >= 200]
  (junction 27) -> (junction 35) [order 2]
  Drive_trip -> (junction 35)
  (junction 35) -> Store_previous_fault [order 1] : [oProp.oMot_.oState_.uiDriveState_ >= 1000]
  (junction 35) -> setTripState [order 2]
  data: oProp data_store_memory; oTilt data_store_memory; iCrossTripTiltToPropulsionMode data_store_memory

== stateflow chart Target_Control_System/MainLoop/tiltMotor_mainLoop/mainTask_tilt/motorTaskMainFastStep(&oTilt)/Software Overcurrent Protection - Tilt/Forced_angle_overcurrent/Chart ==
  state Start
    // During forced angle start use a lower overcurrent limit, because we know exactly how much current should flow in the motor
    entry:
    fMaximumCurrent = oTilt.oMot_.oParam_.fForcedAngleIRef_ * oTilt.oMot_.oParam_.fForcedAngleStartOvercurrentRatio_;
  state Drive_trip
    // Disable the drive and enter a trip state (error state)
    entry:
    oTilt.oMot_.oOut_.uiEnableGateDrive_ = 0;
    oTilt.oMot_.oOut_.uiCurrentControllerActive_ = 0;
    // NOTE: the actual turning off is done in the ctrl interrupt
    // formerly: Xil_Out32(uiGateDriverBaseaddr_, 0x0);
  state Store_previous_fault
    // If we were already in a fault state, store the previous fault:
    entry:
    oTilt.oMot_.oOut_.uiLastFaultState_ = oTilt.oMot_.oState_.uiDriveState_;
  state setTripState
    entry:
    oTilt.oMot_.oState_.uiDriveState_ = 1041;
  (default) -> Start
  Start -> (junction 7) : [single(fabs(oTilt.oMot_.oIn_.oAdcData_.fIa_)) > fMaximumCurrent || ...
      | single(fabs(oTilt.oMot_.oIn_.oAdcData_.fIb_)) > fMaximumCurrent || ...
      | single(fabs(oTilt.oMot_.oIn_.oAdcData_.fIc_)) > fMaximumCurrent]
  setTripState -> Start
  (junction 7) -> Drive_trip [order 1] : [oTilt.oMot_.oState_.uiDriveState_ >= 200]
  (junction 7) -> (junction 14) [order 2]
  Drive_trip -> (junction 14)
  (junction 14) -> Store_previous_fault [order 1] : [oTilt.oMot_.oState_.uiDriveState_ >= 1000]
  (junction 14) -> setTripState [order 2]
  Store_previous_fault -> setTripState
  data: oTilt data_store_memory; fMaximumCurrent local double

== stateflow chart Target_Control_System/MainLoop/tiltMotor_mainLoop/mainTask_tilt/motorTaskMainFastStep(&oTilt)/Software Overcurrent Protection - Tilt/checkForHwOvercurrents(&oTilt)/checkForHwOvercurrents  ==
  state Start
  state setTripState3
    //default aux trip
    entry:
    oTilt.oMot_.oState_.uiDriveState_ = 1018;
  state Drive_trip1
    // Disable the drive and enter a trip state (error state)
    entry:
    oTilt.oMot_.oOut_.uiEnableGateDrive_ = 0;
    oTilt.oMot_.oOut_.uiCurrentControllerActive_ = 0;
    // NOTE: the actual turning off is done in the ctrl interrupt
    // formerly: Xil_Out32(uiGateDriverBaseaddr_, 0x0);
  state Store_previous_fault3
    // If we were already in a fault state, store the previous fault:
    entry:
    oTilt.oMot_.oOut_.uiLastFaultState_ = oTilt.oMot_.oState_.uiDriveState_;
  state Store_previous_fault1
    // If we were already in a fault state, store the previous fault:
    entry:
    oTilt.oMot_.oOut_.uiLastFaultState_ = oTilt.oMot_.oState_.uiDriveState_;
  state Drive_trip3
    // Disable the drive and enter a trip state (error state)
    entry:
    oTilt.oMot_.oOut_.uiEnableGateDrive_ = 0;
    oTilt.oMot_.oOut_.uiCurrentControllerActive_ = 0;
    // NOTE: the actual turning off is done in the ctrl interrupt
    // formerly: Xil_Out32(uiGateDriverBaseaddr_, 0x0);
  state setTripState1
    // Hardware overcurrent trip
    entry:
    oTilt.oMot_.oState_.uiDriveState_ = 1008;
  state Aux_trip
    // Auxiliary trip, one-hot encoding in bits 6:4
    entry:
    oTilt.oMot_.oOut_.uiGateDriverStatus_ &= 0x70;
    fTemp = oTilt.oMot_.oOut_.uiGateDriverStatus_ >> 4;
    oTilt.oMot_.oOut_.uiGateDriverStatus_ = fTemp;
  state Drive_trip2
    // Disable the drive and enter a trip state (error state)
    entry:
    oTilt.oMot_.oOut_.uiEnableGateDrive_ = 0;
    oTilt.oMot_.oOut_.uiCurrentControllerActive_ = 0;
    // NOTE: the actual turning off is done in the ctrl interrupt
    // formerly: Xil_Out32(uiGateDriverBaseaddr_, 0x0);
  state Aux_trip_2
    // Aux trip 2: The hardware monitor for the control voltages has tripped.
    // This circuit is not present on the January 2019 inverters, but the FPGA image holds
    // the lines at the non-tripped levels.
    // Some of the GPIO pins will tell us which voltage rail tripped:
    entry:
    fTemp2 = mdl_tilt_uiFlags & 0x1F;
    fTemp2 ^= 0x4;
    mdl_tilt_uiFlags = fTemp2;
    //3V = 1036; 5V = 1037; 12V = 1038; default = 1039 (more than one control voltage low simultaneously);
  state Store_previous_fault2
    // If we were already in a fault state, store the previous fault:
    entry:
    oTilt.oMot_.oOut_.uiLastFaultState_ = oTilt.oMot_.oState_.uiDriveState_;
  state Drive_trip5
    // Disable the drive and enter a trip state (error state)
    entry:
    oTilt.oMot_.oOut_.uiEnableGateDrive_ = 0;
    oTilt.oMot_.oOut_.uiCurrentControllerActive_ = 0;
    // NOTE: the actual turning off is done in the ctrl interrupt
    // formerly: Xil_Out32(uiGateDriverBaseaddr_, 0x0);
  state setTripState2
    //Aux trip 1: software watchdog timer
    entry:
    oTilt.oMot_.oState_.uiDriveState_ = 1015;
  state Store_previous_fault5
    // If we were already in a fault state, store the previous fault:
    entry:
    oTilt.oMot_.oOut_.uiLastFaultState_ = oTilt.oMot_.oState_.uiDriveState_;
  state Drive_trip4
    // Disable the drive and enter a trip state (error state)
    entry:
    oTilt.oMot_.oOut_.uiEnableGateDrive_ = 0;
    oTilt.oMot_.oOut_.uiCurrentControllerActive_ = 0;
    // NOTE: the actual turning off is done in the ctrl interrupt
    // formerly: Xil_Out32(uiGateDriverBaseaddr_, 0x0);
  state setTripState5
    entry:
    oTilt.oMot_.oState_.uiDriveState_ = aux3_tripCode;
  state Store_previous_fault4
    // If we were already in a fault state, store the previous fault:
    entry:
    oTilt.oMot_.oOut_.uiLastFaultState_ = oTilt.oMot_.oState_.uiDriveState_;
  state setTripState4
    //Aux trip 1: software watchdog timer
    entry:
    oTilt.oMot_.oState_.uiDriveState_ = aux2_tripCode;
  (default) -> Start
  setTripState4 -> Start
  setTripState2 -> Start
  setTripState3 -> Start
  Start -> Aux_trip [order 2] : [(oTilt.oMot_.oOut_.uiGateDriverStatus_ & 0x70) > 0]
  Start -> (junction 20) [order 1] : [(oTilt.oMot_.oOut_.uiGateDriverStatus_ & 0xE) > 0]
  setTripState1 -> Start
  setTripState5 -> Start
  (junction 20) -> Drive_trip1 [order 1] : [oTilt.oMot_.oState_.uiDriveState_ >= 200]
  Store_previous_fault3 -> setTripState3
  (junction 64) -> setTripState3 [order 2]
  (junction 20) -> (junction 25) [order 2]
  Drive_trip1 -> (junction 25)
  (junction 64) -> Store_previous_fault3 [order 1] : [oTilt.oMot_.oState_.uiDriveState_ >= 1000]
  Drive_trip3 -> (junction 64)
  (junction 57) -> (junction 64) [order 2]
  (junction 25) -> Store_previous_fault1 [order 1] : [oTilt.oMot_.oState_.uiDriveState_ >= 1000]
  (junction 25) -> setTripState1 [order 2]
  Store_previous_fault1 -> setTripState1
  (junction 57) -> Drive_trip3 [order 1] : [oTilt.oMot_.oState_.uiDriveState_ >= 200]
  Aux_trip -> (junction 57) [order 4]
  Aux_trip -> (junction 40) [order 3] : [fTemp == 1]
  Aux_trip -> Aux_trip_2 [order 2] : [fTemp == 2]
      | // C code uses oPitch.oMot_.oOut_.uiGateDriverStatus_ == 2, but this value gets rewritten
      | // at each time step so it doesn't work for stateflow transition.
  Aux_trip -> (junction 170) [order 1] : [fTemp == 4]
      | // Aux Trip 3. This is the auxiliary protection unit.
      | // If this is a known error, set that specific fault code.
  (junction 40) -> Drive_trip2 [order 1] : [oTilt.oMot_.oState_.uiDriveState_ >= 200]
  (junction 40) -> (junction 48) [order 2]
  Drive_trip2 -> (junction 48)
  Aux_trip_2 -> (junction 85) [order 1] : [fTemp2 == 1]
      | {aux2_tripCode = 1036;}
  Aux_trip_2 -> (junction 85) [order 2] : [fTemp2 == 2 || ...
      | fTemp2 == 8]
      | {aux2_tripCode = 1037;}
  Aux_trip_2 -> (junction 85) [order 3] : [fTemp2 == 4 || ...
      | fTemp2 == 16]
      | {aux2_tripCode = 1038;}
  Aux_trip_2 -> (junction 85) [order 4] : {aux2_tripCode = 1039;}
  (junction 48) -> Store_previous_fault2 [order 1] : [oTilt.oMot_.oState_.uiDriveState_ >= 1000]
  (junction 48) -> setTripState2 [order 2]
  (junction 170) -> (junction 150) [order 3] : {aux3_tripCode = 1017;}
  Store_previous_fault2 -> setTripState2
  (junction 170) -> (junction 150) [order 2] : [mdl_tilt_uiAPUFlags == 2]
      | {aux3_tripCode = 1035;}
      | // Digitally stuck sensor
  (junction 150) -> Drive_trip5 [order 1] : [oTilt.oMot_.oState_.uiDriveState_ >= 200]
  (junction 170) -> (junction 150) [order 1] : [mdl_tilt_uiAPUFlags == 1]
      | {aux3_tripCode = 1034;}
      | // Phase current sum out of bounds.
      | // This could happen at boot due to offsets.
      | // If this is indeed the case, this fault may
      | // need to be ignored until current zeroing
      | // has been done. For now, keep it simple.
  (junction 150) -> (junction 159) [order 2]
  Drive_trip5 -> (junction 159)
  (junction 159) -> Store_previous_fault5 [order 1] : [oTilt.oMot_.oState_.uiDriveState_ >= 1000]
  (junction 159) -> setTripState5 [order 2]
  (junction 85) -> Drive_trip4 [order 1] : [oTilt.oMot_.oState_.uiDriveState_ >= 200]
  (junction 85) -> (junction 103) [order 2]
  Store_previous_fault5 -> setTripState5
  Drive_trip4 -> (junction 103)
  (junction 103) -> Store_previous_fault4 [order 1] : [oTilt.oMot_.oState_.uiDriveState_ >= 1000]
  (junction 103) -> setTripState4 [order 2]
  Store_previous_fault4 -> setTripState4
  data: aux2_tripCode local single; fTemp local uint32; oTilt data_store_memory; mdl_tilt_uiFlags data_store_memory; aux3_tripCode local double; mdl_tilt_uiAPUFlags data_store_memory; fTemp2 local double
